simulink model "Complete_schema"  (R2014b)
settings: Solver=ode45  StartTime=0.0  StopTime=T_sim  RelTol=1e-3
values from neighbouring files (symbols this model uses):
  Kdlqr_simulink = Kdlqr    [cessna.m]
  N = 10    [cessna.m]
  Q_simulink = Q    [cessna.m]
  R = 10    [cessna.m]
  S_simulink = S    [cessna.m]
  set_point = [0; 0; 0; 0]    [cessna.m]
  sys_discrete = c2d(sys, Ts)    [cessna.m]
  sys_observer_discrete = sys_observer    [cessna.m]
  Ts = 0.1    [cessna.m]
  u_max_simulink = u_max    (= 0.262)    [cessna.m]
  u_min_simulink = u_min    (= -0.262)    [cessna.m]
  uslopemax_simulink = u_slew_rate_max    (= 0.524)    [cessna.m]
  uslopemin_simulink = u_slew_rate_min    (= -0.524)    [cessna.m]
  x0 = [0; 0; 0; 10]    [cessna.m]
  x_max_simulink = [+inf, x2_max, +inf, inf]'    [cessna.m]
  x_min_simulink = [-inf, x2_min, -inf, - inf]'    [cessna.m]
undefined symbols (not defined in the file or in its folder): MPC_controller
settings Model: Creator=lele  LastModifiedBy=lele

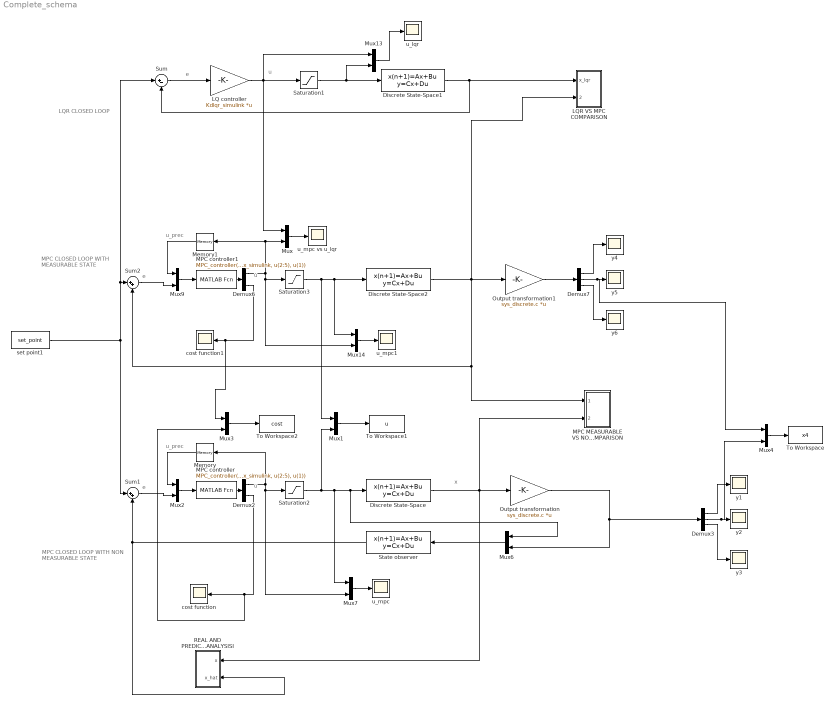
== system Complete_schema ==
  note: MPC CLOSED LOOP WITH NON MEASURABLE STATE
  note: MPC CLOSED LOOP WITH MEASURABLE STATE
  note: LQR CLOSED LOOP
  note: x
  note: u_prec
  note: u
  note: e
  note: u_prec
  note: u
  note: e
  note: u
  note: e
  Demux2 : Demux  Outputs=2
  Demux3 : Demux  Outputs=3
  Demux6 : Demux  Outputs=2
  Demux7 : Demux  Outputs=3
  Discrete State-Space : DiscreteStateSpace  A=sys_discrete.a  B=sys_discrete.b  C=eye(4)  D=zeros(4, 1)  X0=x0  SampleTime=Ts
  Discrete State-Space1 : DiscreteStateSpace  A=sys_discrete.a  B=sys_discrete.b  C=eye(4)  D=zeros(4, 1)  X0=x0  SampleTime=Ts
  Discrete State-Space2 : DiscreteStateSpace  A=sys_discrete.a  B=sys_discrete.b  C=eye(4)  D=zeros(4, 1)  X0=x0  SampleTime=Ts
  LQ controller : Gain  Gain=Kdlqr_simulink  Multiplication=Matrix(K*u)
  LQR VS MPC COMPARISON : Subsystem
  "MPC MEASURABLE VS NON MEASURABLE STATE COMPARISON " : Subsystem
  MPC controller : MATLABFcn  MATLABFcn=MPC_controller(sys_discrete, Q_simulink, R, S_simulink, N, u_min_simulink, u_max_simulink, uslopemin_simulink, uslopemax_simulink, x_min_simulink, x_max_simulink, u(2:5), u(1))  OutputDimensions=2  Output1D=off
  MPC controller1 : MATLABFcn  MATLABFcn=MPC_controller(sys_discrete, Q_simulink, R, S_simulink, N, u_min_simulink, u_max_simulink, uslopemin_simulink, uslopemax_simulink, x_min_simulink, x_max_simulink, u(2:5), u(1))  OutputDimensions=2  Output1D=off
  Memory : Memory
  Memory1 : Memory
  Mux{,1,3..4,6..7,13..14} (8 alike) : Mux  Inputs=2
  Mux2 : Mux  Inputs=[1 4]
  Mux9 : Mux  Inputs=[1 4]
  Output transformation : Gain  Gain=sys_discrete.c  Multiplication=Matrix(K*u)
  Output transformation1 : Gain  Gain=sys_discrete.c  Multiplication=Matrix(K*u)
  REAL AND PREDICTED STATE ANALYSISI : Subsystem
  Saturation1 : Saturate  UpperLimit=u_max_simulink  LowerLimit=u_min_simulink
  Saturation2 : Saturate  UpperLimit=u_max_simulink  LowerLimit=u_min_simulink
  Saturation3 : Saturate  UpperLimit=u_max_simulink  LowerLimit=u_min_simulink
  State observer : DiscreteStateSpace  A=sys_observer_discrete.a  B=sys_observer_discrete.b  C=sys_observer_discrete.c  D=sys_observer_discrete.d  X0=x0  SampleTime=Ts
  Sum : Sum  Inputs=|+-
  Sum1 : Sum  Inputs=|++
  Sum2 : Sum  Inputs=|++
  To Workspace : ToWorkspace  VariableName=x4  SaveFormat=Timeseries  SampleTime=-1
  To Workspace1 : ToWorkspace  VariableName=u  SaveFormat=Timeseries  SampleTime=-1
  To Workspace2 : ToWorkspace  VariableName=cost  SaveFormat=Timeseries  SampleTime=-1
  cost function : Scope
      settings: ShowLegends=on  TimeRange=10  YMin=0  YMax=0.003  SaveName=ScopeData4
  cost function1 : Scope
      settings: ShowLegends=on  YMin=0  YMax=0.003  SaveName=ScopeData13
  set point1 : Constant  Value=set_point
  u_lqr : Scope
      settings: ShowLegends=on
  u_mpc : Scope
      settings: ShowLegends=on  SaveName=ScopeData2
  "u_mpc vs u_lqr " : Scope
      settings: ShowLegends=on  SaveName=ScopeData3
  u_mpc1 : Scope
      settings: ShowLegends=on  SaveName=ScopeData14
  y{1..6} (6 alike) : Scope
      y1 settings: ShowLegends=on  SaveName=ScopeData10
      y2 settings: ShowLegends=on  SaveName=ScopeData11
      y3 settings: ShowLegends=on  SaveName=ScopeData12
      y4 settings: ShowLegends=on  SaveName=ScopeData19
      y5 settings: ShowLegends=on  SaveName=ScopeData20
      y6 settings: ShowLegends=on  SaveName=ScopeData21
  wires:
  Sum1/1 -> Mux2/2
  Mux2/1 -> MPC controller/1
  Memory/1 -> Mux2/1
  Saturation2/1 -> Mux1/2, Mux7/1, Mux6/1, Discrete State-Space/1
  Mux7/1 -> u_mpc/1
  MPC controller/1 -> Demux2/1
  Demux2/1 -> Mux7/2, Saturation2/1, Memory/1
  Demux2/2 -> Mux3/2, cost function/1
  Output transformation/1 -> Mux6/2, Demux3/1
  Demux3/1 -> y1/1
  Demux3/2 -> Mux4/2, y2/1
  Demux3/3 -> y3/1
  Discrete State-Space/1 -> "MPC MEASURABLE VS NON MEASURABLE STATE COMPARISON "/2(x_mpc_nonmeasurable), REAL AND PREDICTED STATE ANALYSISI/1(x), Output transformation/1
  State observer/1 -> REAL AND PREDICTED STATE ANALYSISI/2(x_hat), Sum1/2
  Mux6/1 -> State observer/1
  set point1/1 -> Sum/1, Sum2/1, Sum1/1
  Sum/1 -> LQ controller/1
  Discrete State-Space1/1 -> Sum/2, LQR VS MPC COMPARISON/1(x_lqr)
  LQ controller/1 -> Mux13/1, Mux/1, Saturation1/1
  Saturation1/1 -> Mux13/2, Discrete State-Space1/1
  Mux/1 -> "u_mpc vs u_lqr "/1
  Sum2/1 -> Mux9/2
  Mux9/1 -> MPC controller1/1
  Memory1/1 -> Mux9/1
  Saturation3/1 -> Mux1/1, Mux14/1, Discrete State-Space2/1
  Mux13/1 -> u_lqr/1
  Mux14/1 -> u_mpc1/1
  MPC controller1/1 -> Demux6/1
  Demux6/1 -> Mux14/2, Saturation3/1, Memory1/1, Mux/2
  Demux6/2 -> Mux3/1, cost function1/1
  Output transformation1/1 -> Demux7/1
  Demux7/1 -> y4/1
  Demux7/2 -> Mux4/1, y5/1
  Demux7/3 -> y6/1
  Discrete State-Space2/1 -> LQR VS MPC COMPARISON/2(x_mpc), "MPC MEASURABLE VS NON MEASURABLE STATE COMPARISON "/1(x_mpc_measurable), Sum2/2, Output transformation1/1
  Mux1/1 -> To Workspace1/1
  Mux3/1 -> To Workspace2/1
  Mux4/1 -> To Workspace/1

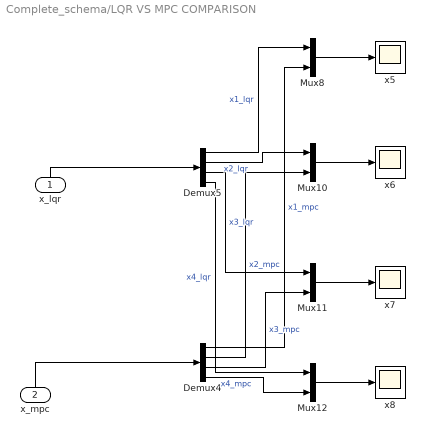
== system Complete_schema/LQR VS MPC COMPARISON ==
  x_lqr : Inport
  x_mpc : Inport  Port=2
  Demux4 : Demux
  Demux5 : Demux
  Mux{8,10..12} (4 alike) : Mux  Inputs=2
  x{5..8} (4 alike) : Scope
      x5 settings: ShowLegends=on  TimeRange=10  SaveName=ScopeData15
      x6 settings: ShowLegends=on  SaveName=ScopeData16
      x7 settings: ShowLegends=on  SaveName=ScopeData17
      x8 settings: ShowLegends=on  SaveName=ScopeData18
  wires:
  Mux11/1 -> x7/1
  Demux4/1 -> Mux8/2  "x1_mpc"
  x_lqr/1 -> Demux5/1
  Demux5/1 -> Mux8/1  "x1_lqr"
  Demux4/3 -> Mux11/2  "x3_mpc"
  Demux5/4 -> Mux12/1  "x4_lqr"
  Demux5/3 -> Mux11/1  "x3_lqr"
  x_mpc/1 -> Demux4/1
  Mux8/1 -> x5/1
  Mux10/1 -> x6/1
  Mux12/1 -> x8/1
  Demux4/4 -> Mux12/2  "x4_mpc"
  Demux4/2 -> Mux10/2  "x2_mpc"
  Demux5/2 -> Mux10/1  "x2_lqr"

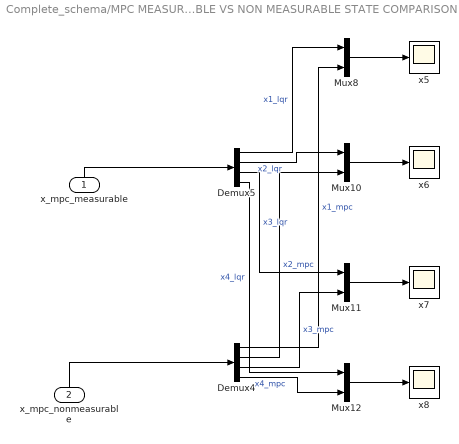
== system Complete_schema/MPC MEASURABLE VS NON MEASURABLE STATE COMPARISON  ==
  x_mpc_measurable : Inport
  x_mpc_nonmeasurable : Inport  Port=2
  Demux4 : Demux
  Demux5 : Demux
  Mux{8,10..12} (4 alike) : Mux  Inputs=2
  x{5..8} (4 alike) : Scope
      x5 settings: ShowLegends=on  TimeRange=10  SaveName=ScopeData15
      x6 settings: ShowLegends=on  SaveName=ScopeData16
      x7 settings: ShowLegends=on  SaveName=ScopeData17
      x8 settings: ShowLegends=on  SaveName=ScopeData18
  wires:
  Mux11/1 -> x7/1
  Demux4/1 -> Mux8/2  "x1_mpc"
  x_mpc_measurable/1 -> Demux5/1
  Demux5/1 -> Mux8/1  "x1_lqr"
  Demux4/3 -> Mux11/2  "x3_mpc"
  Demux5/4 -> Mux12/1  "x4_lqr"
  Demux5/3 -> Mux11/1  "x3_lqr"
  x_mpc_nonmeasurable/1 -> Demux4/1
  Mux8/1 -> x5/1
  Mux10/1 -> x6/1
  Mux12/1 -> x8/1
  Demux4/4 -> Mux12/2  "x4_mpc"
  Demux4/2 -> Mux10/2  "x2_mpc"
  Demux5/2 -> Mux10/1  "x2_lqr"

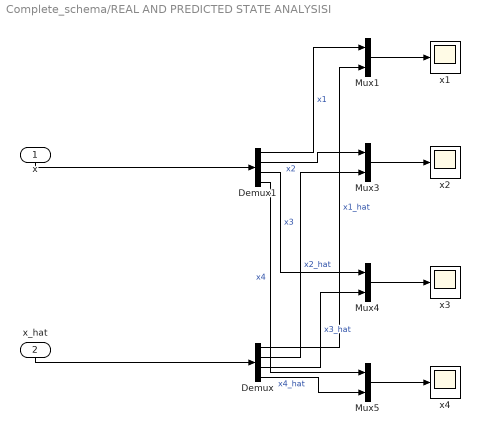
== system Complete_schema/REAL AND PREDICTED STATE ANALYSISI ==
  x : Inport
  x_hat : Inport  Port=2
  Demux : Demux
  Demux1 : Demux
  Mux{1,3..5} (4 alike) : Mux  Inputs=2
  x{1..4} (4 alike) : Scope
      x1 settings: ShowLegends=on  TimeRange=10  SaveName=ScopeData6
      x2 settings: ShowLegends=on  SaveName=ScopeData7
      x3 settings: ShowLegends=on  SaveName=ScopeData8
      x4 settings: ShowLegends=on  YMin=-3  YMax=6  SaveName=ScopeData9
  wires:
  Demux1/2 -> Mux3/1  "x2"
  Mux5/1 -> x4/1
  Mux1/1 -> x1/1
  Demux1/3 -> Mux4/1  "x3"
  Demux/4 -> Mux5/2  "x4_hat"
  Mux4/1 -> x3/1
  Demux/2 -> Mux3/2  "x2_hat"
  x/1 -> Demux1/1
  Mux3/1 -> x2/1
  Demux/3 -> Mux4/2  "x3_hat"
  Demux1/1 -> Mux1/1  "x1"
  Demux/1 -> Mux1/2  "x1_hat"
  Demux1/4 -> Mux5/1  "x4"
  x_hat/1 -> Demux/1
